simulink model "PWMGenerator"  (R2022a)
settings: Solver=VariableStepAuto  StartTime=0.0  StopTime=0.8  MaxStep=1e-6  RelTol=1e-3
libraries: spsTriangleGeneratorLib x2
settings Model: Creator=sebastian  LastModifiedBy=sebastian

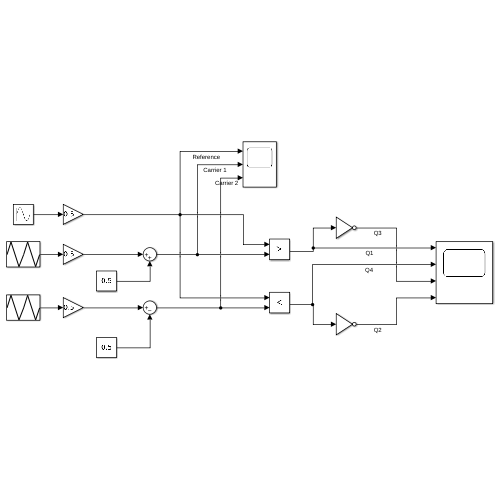
[thumbnail: Simulink's stored preview of the top-level diagram]
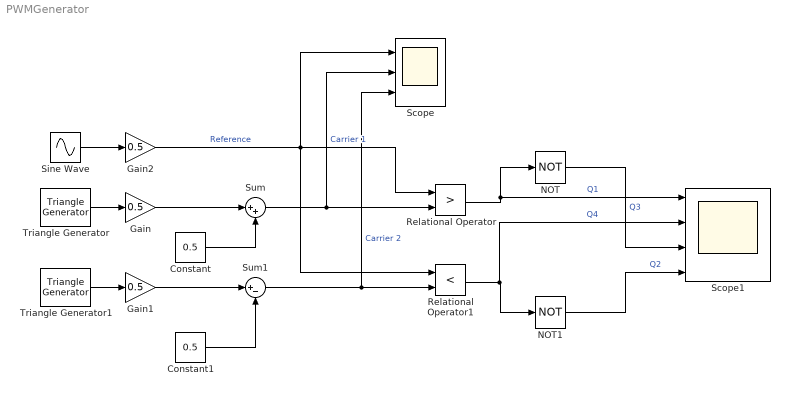
== system PWMGenerator ==
  Constant : Constant  Value=0.5
  Constant1 : Constant  Value=0.5
  Gain : Gain  Gain=0.5
  Gain1 : Gain  Gain=0.5
  Gain2 : Gain  Gain=0.5
  NOT : Logic  Operator=NOT  IconShape=distinctive  AllPortsSameDT=off  OutDataTypeStr=boolean
  NOT1 : Logic  Operator=NOT  IconShape=distinctive  AllPortsSameDT=off  OutDataTypeStr=boolean
  Relational Operator : RelationalOperator  Operator=>  OutDataTypeStr=boolean  RndMeth=Simplest  InputSameDT=off
  Relational Operator1 : RelationalOperator  Operator=<  OutDataTypeStr=boolean  RndMeth=Simplest  InputSameDT=off
  Scope : Scope  NumInputPorts=3
  Scope1 : Scope  NumInputPorts=4
  Sine Wave : Sin  Frequency=10  SampleTime=0
  Sum : Sum  Inputs=|++
  Sum1 : Sum  Inputs=|+-
  Triangle Generator : spsTriangleGeneratorLib/Triangle Generator  Freq=100  Phase=90  Ts=0
  Triangle Generator1 : spsTriangleGeneratorLib/Triangle Generator  Freq=100  Phase=90  Ts=0
  wires:
  Gain/1 -> Sum/1
  Constant/1 -> Sum/2
  Sine Wave/1 -> Gain2/1
  Sum/1 -> Relational Operator/2, Scope/2  "Carrier 1"
  Triangle Generator/1 -> Gain/1
  Triangle Generator1/1 -> Gain1/1
  Gain1/1 -> Sum1/1
  Constant1/1 -> Sum1/2
  Sum1/1 -> Relational Operator1/2, Scope/3  "Carrier 2"
  Relational Operator/1 -> Scope1/1, NOT/1  "Q1"
  Relational Operator1/1 -> Scope1/2, NOT1/1  "Q4"
  NOT1/1 -> Scope1/4  "Q2"
  NOT/1 -> Scope1/3  "Q3"
  Gain2/1 -> Relational Operator1/1, Scope/1, Relational Operator/1  "Reference"
